simulink model "line_lateral_system_simulink"  (R2025b)
settings: Solver=ode45  StartTime=0.0  StopTime=10.0  RelTol=1e-3
libraries: simulink x1
settings Model: Creator=ganes  LastModifiedBy=ganes

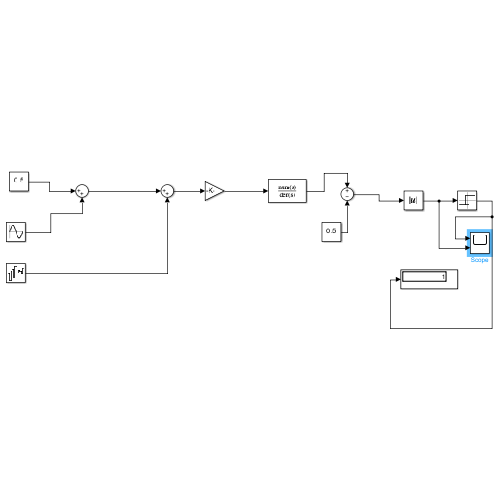
[thumbnail: Simulink's stored preview of the top-level diagram]
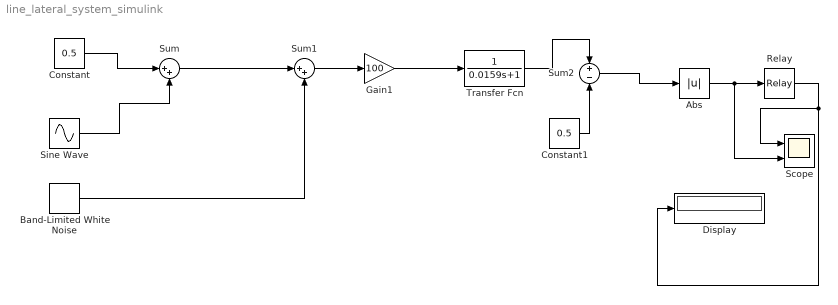
== system line_lateral_system_simulink ==
  Abs : Abs  SaturateOnIntegerOverflow=off
  Band-Limited White Noise : simulink/Sources/Band-Limited White Noise  Cov=0.001  Ts=0.01  seed=[23341]
  Constant : Constant  Value=0.5
  Constant1 : Constant  Value=0.5
  Display : Display
  Gain1 : Gain  Gain=100
  Relay : Relay  OnSwitchValue=0.15  OffSwitchValue=0.10
  Scope : Scope  NumInputPorts=2
      settings: ActiveDisplayYMinimum=-8.3660240740617269  ActiveDisplayYMaximum=136.76138449242455
  Sine Wave : Sin  Amplitude=0.2  Frequency=12.566  SampleTime=0
  Sum : Sum  Inputs=|++
  Sum1 : Sum  Inputs=|++
  Sum2 : Sum  Inputs=+-
  Transfer Fcn : TransferFcn  Denominator=[0.0159 1]
  wires:
  Constant/1 -> Sum/1
  Sine Wave/1 -> Sum/2
  Sum/1 -> Sum1/1
  Band-Limited White Noise/1 -> Sum1/2
  Sum1/1 -> Gain1/1
  Gain1/1 -> Transfer Fcn/1
  Transfer Fcn/1 -> Sum2/1
  Constant1/1 -> Sum2/2
  Sum2/1 -> Abs/1
  Abs/1 -> Scope/2, Relay/1
  Relay/1 -> Display/1, Scope/1
